simulink library "family_6_variant_2_AR_Drone_2_Library"  (R2014b)
settings: Solver=ode45  StartTime=0.0  StopTime=10.0  RelTol=1e-3
libraries: simulink x5, Navigation_KF_Lib x1, Navigation_Lib x1
settings Model: Creator=darenlee  LastModifiedBy=Raphaël

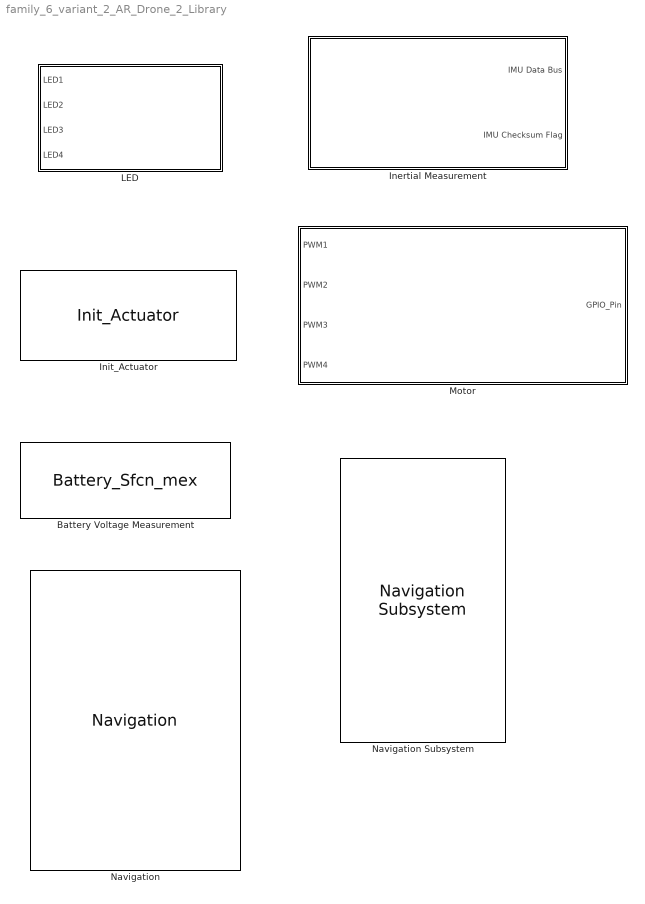
== system family_6_variant_2_AR_Drone_2_Library ==
  Battery Voltage Measurement : S-Function  FunctionName=Battery_Sfcn_mex  Parameters=SampleTime  EnableBusSupport=off  mask(Read Battery Voltage){SFunctionSpec=void BatteryMeasure_step(single y1[1]), SampleTime=-1}
      mask prompts: SampleTime "Sample time (-1 for inherited):"
      mask help:
      | Using I2C, this block reads Battery Voltage from ADCIN0 on the AR Drone 2.0's main board.
      |
      | From reading raw ADC values, one can observe a a linear response
      | 9.0V=662, 9.5V=698, 10.0V=737,10.5V=774, 11.0V=811, 11.5V=848, 12.0V=886, 12.5V=923
      | This leads to our 0.13595166 magic number for decivolts conversion, which the raw ADC
      | value gets multiplied internally.
      |
      | To convert to regular voltage (V) units, multiply the output of this block by 10.
      mask Display: fprintf('Battery Voltage Measurement');
  Inertial Measurement : Subsystem  mask{Ts=1/400}
      mask help: The ARM Cortex A9 SOC connects to this navigation board (PIC16 Microcontroller) over a serial cable connection. This has already been connected by default. The PIC microcontroller reads in sensor data which will handle the ADC readings. One thing to note is that the IMU board controlled by the PIC microcontroller operates at 200 Hz. If this block is set to a sample rate below that, it has been noted that packets will occasionally drop, especially in External Mode. To that end, it is better to sample this block at a higher sample rate above 200 Hz such that we do not get fragmented data packets. If the sample rate is too low the data might become fragmented and will consider that a 'lost' packet
      mask Help:
      | The ARM Cortex A9 SOC connects to this navigation board (PIC16 Microcontroller) over a serial cable connection. This has already been connected by default. The PIC microcontroller reads in sensor data which will handle the ADC readings. One thing to note is that the IMU board controlled by the PIC microcontroller operates at 200 Hz. If this block is set to a sample rate below that, it has been noted that packets will occasionally drop, especially in External Mode. To that end, it is better to sample this block at a higher sample rate above 200 Hz such that we do not get fragmented data packets. If the sample rate is too low the data might become fragmented and will consider that a 'lost' packet
      | 
      | The complete navigation 'struct' or bus signal looks like this:
      | 
      |  typedef struct  __attribute__ ((packed)){
      |         uint16_t taille;
      |         uint16_t nu_trame;
      | 
      |         uint16_t ax;
      |         uint16_t ay;
      |         uint16_t az;
      | 
      |         int16_t vx;
      |         int16_t vy;
      |         int16_t vz;
      |         uint16_t temperature_acc;
      |         uint16_t temperature_gyro;
      | 
      |         uint16_t ultrasound;
      | 
      |         uint16_t us_debut_echo;
      |         uint16_t us_fin_echo;
      |         uint16_t us_association_echo;
      |         uint16_t us_distance_echo;
      | 
      |         uint16_t us_curve_time;
      |         uint16_t us_curve_value;
      |         uint16_t us_curve_ref;
      | 
      |         uint16_t nb_echo;
      | 
      |         uint32_t sum_echo; //unsigned long
      |         int16_t gradient;
      | 
      |         uint16_t flag_echo_ini;
      | 
      |         int32_t pressure;
      |         uint16_t temperature_pressure;
      | 
      |         int16_t my;
      |         int16_t mx;
      |         int16_t mz;
      | 
      |         uint16_t chksum;
      | 
      |     }IMU_Packets;
      mask DialogControl DescGroupVar Prompt: Inertial Measurement Unit Block
      mask DialogControl DescTextVar Prompt: This block will output a bus signal containing data directly from the Inertial Measurement Unit board. The four major measurements include 3-axis sensors readings of the Rate Gyro, Accelerometer, Magnetometer. A scalar ultrasound altimeter reading provides relative distance to the ground. The IMU data bus includes many other readings include barometer, temperature sensing and a wide range of other sensor readings
      mask DialogControl Control3 Prompt: The ARM Cortex A9 SOC connects to this navigation board (PIC16 Microcontroller) over a serial cable connection. This has already been connected by default. The PIC microcontroller reads in sensor data which will handle the ADC readings. One thing to note is that the IMU board controlled by the PIC microcontroller operates at 200 Hz. If this block is set to a sample rate below that, it has been noted that packets will occasionally drop, especially in External Mode. To that end, it is better to sample this block at a higher sample rate above 200 Hz such that we do not get fragmented data packets. If the sample rate is too low the data might become fragmented and will consider that a 'lost' packet
      mask DialogControl Control5 Prompt: A checksum flag output has been provided to indicate when the checksum fails, which can be attributed to packet loss.
      mask DialogControl Control2 Prompt: Sample Time
      mask DialogControl Load_Bus_Obj Prompt: Load Navigation Bus Object From Library
      mask DialogControl Load_Bus_Obj Callback:
      | LibPath = which('AR_Drone_2_Library');
      | MagicValue = regexp(LibPath,'AR_Drone_2_Library.slx');
      | 
      | load([LibPath(1:(MagicValue-1)) 'Save_IMU_struct.mat'])
      | clear LibPath;
      | clear MagicValue;
      mask Display:
      | fprintf('Rate Gyro \n Accelerometer \n Magnetometer \n Ultrasound Altimeter')
      | port_label('output',1,'IMU Data Bus')
      | port_label('output',2,'IMU Checksum Flag')
  Init_Actuator : S-Function  FunctionName=Init_Actuator  EnableBusSupport=off  mask{SFunctionSpec=, ShowSpec=on}
      mask prompts: ShowSpec "Display function specification"
      mask help: This block must be placed in the Simulink model to be able to use the motor actuator and LED blocks
      mask Callback ShowSpec:
      | if strcmp(get_param(gcbh, 'ShowSpec'), 'on')
      |   set_param(gcbh, 'MaskDisplay', sprintf('fprintf(''%s'');', get_param(gcbh, 'SFunctionSpec')));
      | else
      |   set_param(gcbh, 'MaskDisplay', sprintf('fprintf(''%s'');', get_param(gcbh, 'FunctionName')));
      | end
      mask Display: fprintf('Initialize Motor and LED Module');
  LED : Subsystem
      mask help:
      | The quadcopter has 4 LEDs, one for each of the motors. The LEDs can emit 3 colours viz. RED, GREEN AND ORANGE. The input to the block are integers from 0-3 and the numbers represent the colours as follows:
      |
      | 0 - OFF
      | 1 - RED
      | 2 - GREEN
      | 3 - ORANGE
      settings: CopyFcn=%check_init_block  DeleteFcn=%clear x  DestroyFcn=%clear x
      mask Display:
      | fprintf('LED Color Input')
      | port_label('input',1,'LED1');
      | port_label('input',2,'LED2');
      | port_label('input',3,'LED3');
      | port_label('input',4,'LED4');
  Motor : Subsystem
      mask help: The quadcopter has 4 rotors. The input to the rotors are PWM values which are percentage of the full speed of the rotor with 0% being no speed and 100% being full speed. The inputs values are limited to this range. The block converts the 4 PWM values into a 40 bit number which is then fed to the motor controller.
      settings: CopyFcn=%check_init_block
      mask Display:
      | fprintf('Propeller Actuation Input');
      | port_label('input',1,'PWM1');
      | port_label('input',2,'PWM2');
      | port_label('input',3,'PWM3');
      | port_label('input',4,'PWM4');
      | port_label('output',1,'GPIO_Fault_Pin');
  Navigation : Navigation_KF_Lib/Navigation
  Navigation Subsystem : Navigation_Lib/Navigation Subsystem  TempProcessVariant=1  PI_YAW_CORRECT=[-0.9 -0.0001]  D_YAW_CORRECT=0  P_GAIN_ROLLPITCH=-2  I_GAIN_ROLLPITCH=-0.01  ACCEL_OFFSET_X=0  ACCEL_OFFSET_Y=0  ACCEL_OFFSET_Z=0

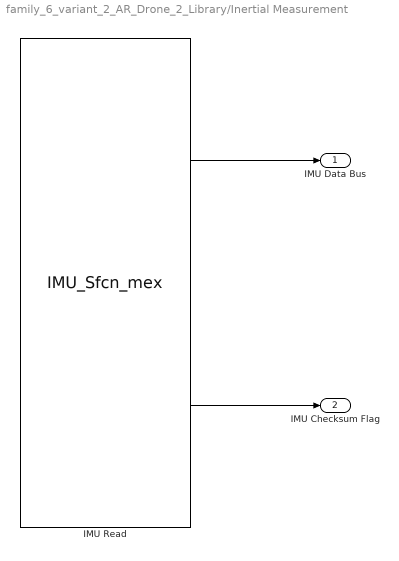
== system family_6_variant_2_AR_Drone_2_Library/Inertial Measurement ==
  IMU Read : S-Function  FunctionName=IMU_Sfcn_mex  Parameters=SampleTime  EnableBusSupport=off  mask(Legacy Function){SFunctionSpec=void MDL_IMU_step(IMU_Packets y1[1], int32 y2[1]), SampleTime=Ts, ShowSpec=on}
      mask prompts: SampleTime "Sample time (-1 for inherited):"; ShowSpec "Display function specification"
      mask help:
      | This block allows you to call the legacy functions specified by the following Legacy Code Tool definition:
      | def.SFunctionName = 'IMU_Sfcn_mex';
      | def.InitializeConditionsFcnSpec = 'void MDL_IMU_start()';
      | def.OutputFcnSpec = 'void MDL_IMU_step(IMU_Packets y1[1], int32 y2[1])';
      | def.TerminateFcnSpec = 'void MDL_IMU_term()';
      | def.SourceFiles = {'IMU_Navdata_Wrapper.c'};
      | def.SampleTime = 'parameterized';
      | def.Options.useTlcWithAccel = false;
      mask Help: <p>This block was generated automatically by the Legacy Code Tool. For detailed help on this tool, call<a href="matlab:legacy_code('help')"> legacy_code('help')</a>.</p>
      mask Callback ShowSpec:
      | if strcmp(get_param(gcbh, 'ShowSpec'), 'on')
      |   set_param(gcbh, 'MaskDisplay', sprintf('fprintf(''%s'');', get_param(gcbh, 'SFunctionSpec')));
      | else
      |   set_param(gcbh, 'MaskDisplay', sprintf('fprintf(''%s'');', get_param(gcbh, 'FunctionName')));
      | end
      mask Display: fprintf('void MDL_IMU_step(IMU_Packets y1[1], int32 y2[1])');
  IMU Data Bus : Outport
  IMU Checksum Flag : Outport  Port=2
  wires:
  IMU Read/2 -> IMU Checksum Flag/1
  IMU Read/1 -> IMU Data Bus/1

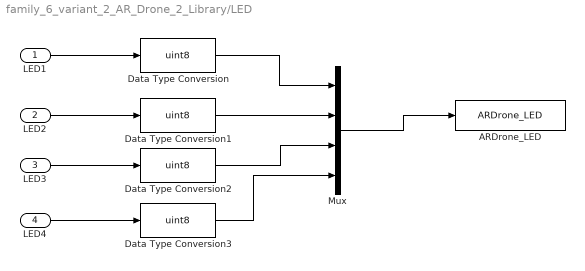
== system family_6_variant_2_AR_Drone_2_Library/LED ==
  LED1 : Inport
  LED2 : Inport  Port=2
  LED3 : Inport  Port=3
  LED4 : Inport  Port=4
  ARDrone_LED : S-Function  FunctionName=ARDrone_LED  EnableBusSupport=off  mask(Legacy Function){SFunctionSpec=LED_set(uint8 u1[4]), ShowSpec=on}
      mask prompts: ShowSpec "Display function specification"
      mask help:
      | This block allows you to call the legacy functions specified by the following Legacy Code Tool definition:
      | def.SFunctionName = 'ARDrone_LED';
      | def.OutputFcnSpec = 'LED_set(uint8 u1[4])';
      | def.HeaderFiles = {'led.h'};
      | def.SourceFiles = {'led.c'};
      | def.IncPaths = {'.'};
      mask Help: <p>This block was generated automatically by the Legacy Code Tool. For detailed help on this tool, call<a href="matlab:legacy_code('help')"> legacy_code('help')</a>.</p>
      mask Callback ShowSpec:
      | if strcmp(get_param(gcbh, 'ShowSpec'), 'on')
      |   set_param(gcbh, 'MaskDisplay', sprintf('fprintf(''%s'');', get_param(gcbh, 'SFunctionSpec')));
      | else
      |   set_param(gcbh, 'MaskDisplay', sprintf('fprintf(''%s'');', get_param(gcbh, 'FunctionName')));
      | end
      mask Display: fprintf('LED_set(uint8 u1[4])');
  Data Type Conversion{,1..3} (4 alike) : DataTypeConversion  OutDataTypeStr=uint8
  Mux : Mux
  wires:
  LED2/1 -> Data Type Conversion1/1
  LED1/1 -> Data Type Conversion/1
  Mux/1 -> ARDrone_LED/1
  LED4/1 -> Data Type Conversion3/1
  Data Type Conversion/1 -> Mux/1
  Data Type Conversion1/1 -> Mux/2
  Data Type Conversion3/1 -> Mux/4
  LED3/1 -> Data Type Conversion2/1
  Data Type Conversion2/1 -> Mux/3

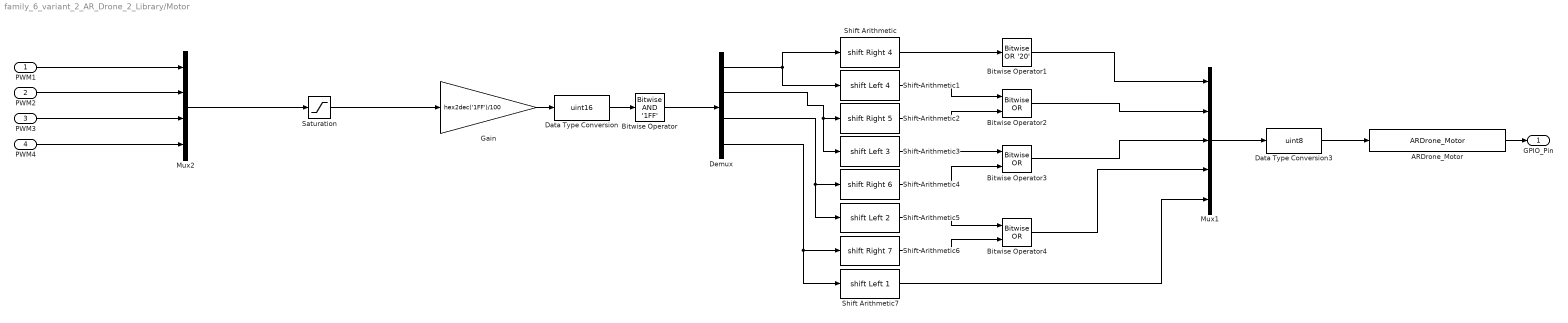
== system family_6_variant_2_AR_Drone_2_Library/Motor ==
  PWM1 : Inport
  PWM2 : Inport  Port=2
  PWM3 : Inport  Port=3
  PWM4 : Inport  Port=4
  ARDrone_Motor : S-Function  FunctionName=ARDrone_Motor  EnableBusSupport=off  mask(Legacy Function){SFunctionSpec=uint16 y1 = Motor_Set(uint8 u1[5]), ShowSpec=on}
      mask prompts: ShowSpec "Display function specification"
      mask help:
      | This block allows you to call the legacy functions specified by the following Legacy Code Tool definition:
      | def.SFunctionName = 'ARDrone_Motor';
      | def.OutputFcnSpec = 'uint16 y1 = Motor_Set(uint8 u1[5])';
      | def.HeaderFiles = {'motor.h'};
      | def.SourceFiles = {'motor.c'};
      | def.IncPaths = {'.'};
      mask Help: <p>This block was generated automatically by the Legacy Code Tool. For detailed help on this tool, call<a href="matlab:legacy_code('help')"> legacy_code('help')</a>.</p>
      mask Callback ShowSpec:
      | if strcmp(get_param(gcbh, 'ShowSpec'), 'on')
      |   set_param(gcbh, 'MaskDisplay', sprintf('fprintf(''%s'');', get_param(gcbh, 'SFunctionSpec')));
      | else
      |   set_param(gcbh, 'MaskDisplay', sprintf('fprintf(''%s'');', get_param(gcbh, 'FunctionName')));
      | end
      mask Display: fprintf('uint16 y1 = Motor_Set(uint8 u1[5])');
  Bitwise Operator : simulink/Logic and Bit Operations/Bitwise Operator  logicop=AND  UseBitMask=on  BitMask='1FF'  BitMaskRealWorld=Stored Integer
  Bitwise Operator1 : simulink/Logic and Bit Operations/Bitwise Operator  logicop=OR  UseBitMask=on  BitMask='20'  BitMaskRealWorld=Stored Integer
  Bitwise Operator2 : simulink/Logic and Bit Operations/Bitwise Operator  logicop=OR  UseBitMask=off  NumInputPorts=2  BitMask='20'  BitMaskRealWorld=Stored Integer
  Bitwise Operator3 : simulink/Logic and Bit Operations/Bitwise Operator  logicop=OR  UseBitMask=off  NumInputPorts=2  BitMask='20'  BitMaskRealWorld=Stored Integer
  Bitwise Operator4 : simulink/Logic and Bit Operations/Bitwise Operator  logicop=OR  UseBitMask=off  NumInputPorts=2  BitMask='20'  BitMaskRealWorld=Stored Integer
  Data Type Conversion : DataTypeConversion  OutDataTypeStr=uint16
  Data Type Conversion3 : DataTypeConversion  OutDataTypeStr=uint8
  Demux : Demux
  Gain : Gain  Gain=hex2dec('1FF')/100
  Mux1 : Mux  Inputs=5
  Mux2 : Mux
  Saturation : Saturate  UpperLimit=100  LowerLimit=0
  Shift Arithmetic : ArithShift  BitShiftNumber=4  BitShiftDirection=Right
  Shift Arithmetic1 : ArithShift  BitShiftNumber=4  BitShiftDirection=Left
  Shift Arithmetic2 : ArithShift  BitShiftNumber=5  BitShiftDirection=Right
  Shift Arithmetic3 : ArithShift  BitShiftNumber=3  BitShiftDirection=Left
  Shift Arithmetic4 : ArithShift  BitShiftNumber=6  BitShiftDirection=Right
  Shift Arithmetic5 : ArithShift  BitShiftNumber=2  BitShiftDirection=Left
  Shift Arithmetic6 : ArithShift  BitShiftNumber=7  BitShiftDirection=Right
  Shift Arithmetic7 : ArithShift  BitShiftNumber=1  BitShiftDirection=Left
  GPIO_Pin : Outport
  wires:
  Data Type Conversion/1 -> Bitwise Operator/1
  Mux1/1 -> Data Type Conversion3/1
  Shift Arithmetic3/1 -> Bitwise Operator3/1
  Shift Arithmetic2/1 -> Bitwise Operator2/2
  Bitwise Operator3/1 -> Mux1/3
  Shift Arithmetic6/1 -> Bitwise Operator4/2
  PWM1/1 -> Mux2/1
  Gain/1 -> Data Type Conversion/1
  Bitwise Operator1/1 -> Mux1/1
  Demux/4 -> Shift Arithmetic7/1, Shift Arithmetic6/1
  Bitwise Operator2/1 -> Mux1/2
  Data Type Conversion3/1 -> ARDrone_Motor/1
  Shift Arithmetic5/1 -> Bitwise Operator4/1
  Demux/2 -> Shift Arithmetic3/1, Shift Arithmetic2/1
  Shift Arithmetic7/1 -> Mux1/5
  PWM4/1 -> Mux2/4
  PWM2/1 -> Mux2/2
  PWM3/1 -> Mux2/3
  Bitwise Operator4/1 -> Mux1/4
  Mux2/1 -> Saturation/1
  Shift Arithmetic/1 -> Bitwise Operator1/1
  Saturation/1 -> Gain/1
  Shift Arithmetic1/1 -> Bitwise Operator2/1
  Bitwise Operator/1 -> Demux/1
  Demux/3 -> Shift Arithmetic5/1, Shift Arithmetic4/1
  Shift Arithmetic4/1 -> Bitwise Operator3/2
  Demux/1 -> Shift Arithmetic/1, Shift Arithmetic1/1
  ARDrone_Motor/1 -> GPIO_Pin/1
